simulink model "COSIM"  (R2017b)
settings: Solver=VariableStepAuto  StartTime=0.0  StopTime=N  RelTol=1e-3
libraries: modelsimlib x1
settings Model: Creator=o_cotte  LastModifiedBy=o_cotte

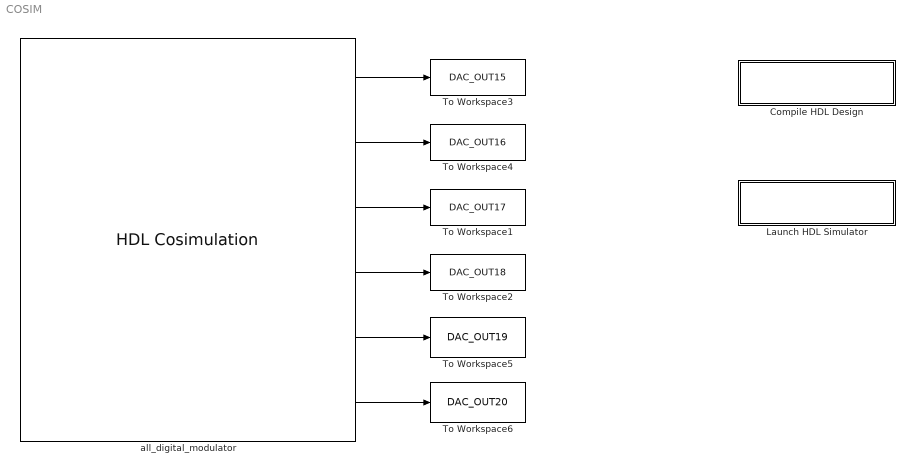
== system COSIM ==
  Compile HDL Design : Subsystem
      settings: OpenFcn=eval('compile_hdl_design_all_digital_modulator');
      mask Display: disp(['Double-Click to' char(10) 'compile HDL files'])
  Launch HDL Simulator : Subsystem
      settings: OpenFcn=eval('launch_hdl_simulator_all_digital_modulator');
      mask Display: disp(['Double-Click to' char(10) 'launch HDL simulator'])
  To Workspace1 : ToWorkspace  VariableName=DAC_OUT17  SampleTime=-1
  To Workspace2 : ToWorkspace  VariableName=DAC_OUT18  SampleTime=-1
  To Workspace3 : ToWorkspace  VariableName=DAC_OUT15  SampleTime=-1
  To Workspace4 : ToWorkspace  VariableName=DAC_OUT16  SampleTime=-1
  To Workspace5 : ToWorkspace  VariableName=DAC_OUT19  SampleTime=-1
  To Workspace6 : ToWorkspace  VariableName=DAC_OUT20  SampleTime=-1
  all_digital_modulator : modelsimlib/HDL Cosimulation  PortPaths=/all_digital_modulator/bypass;/all_digital_modulator/DAC_IN;/all_digital_modulator/DAC_OUT;/all_digital_modulator/DAC_OUT1;/all_digital_modulator/DAC_OUT2;/all_digital_modulator/DAC_OUT3;/all_digital_modulator/DAC_OUT4;/all_digital_modulator/DAC_OUT5;  PortModes=[1 1 2 2 2 2 2 2 ]  PortTimes=[-1,-1,1,1,1,1,1,1]  PortSigns=[-1,-1,1,1,1,1,1,1,]  PortFracLengths=[0,0,32,32,32,32,32,32]  CommLocal=on  CommSharedMemory=off  CommPortNumber=51181  CommShowInfo=on  ClockModes=[]  ClockTimes=[]  TclPreSimCommand=|  TclPostSimCommand=|  TimingMode=ns  TimingScaleFactor=1  idxCellArray={'UNUSED_VAR'}  CosimBypass=Full Simulation  AllowDirectFeedthrough=on  ProductName=EDA Simulator Link MQ  RunAutoTimescale=off  HdlClocks=/all_digital_modulator/sys_clk 32.552 ns;  PreRunTime=130.208  PreRunTimeUnit=ns
      TclPreSimCommand=|
      | force /all_digital_modulator/sys_clk 0 0 ns, 1 16.276 ns -repeat 32.552 ns;
      | force /all_digital_modulator/sys_rst_n 0 0 ns, 1 100 ns;
      TclPostSimCommand=|
      | noforce /all_digital_modulator/sys_clk;
      | noforce /all_digital_modulator/sys_rst_n;
      | puts "done";
      settings: SourceProductName=HDL Verifier
  wires:
  all_digital_modulator/1 -> To Workspace3/1
  all_digital_modulator/5 -> To Workspace5/1
  all_digital_modulator/6 -> To Workspace6/1
  all_digital_modulator/4 -> To Workspace2/1
  all_digital_modulator/3 -> To Workspace1/1
  all_digital_modulator/2 -> To Workspace4/1

== system COSIM/Compile HDL Design ==

== system COSIM/Launch HDL Simulator ==
